simulink model "es1_catena_chiusa_2"  (R2014a)
settings: Solver=ode45  StartTime=0.0  StopTime=20.0  RelTol=1e-3
values from neighbouring files (symbols this model uses):
  Kc = 5    [es1.m]
libraries: cstblocks x2
settings Model: Creator=HP  LastModifiedBy=HP

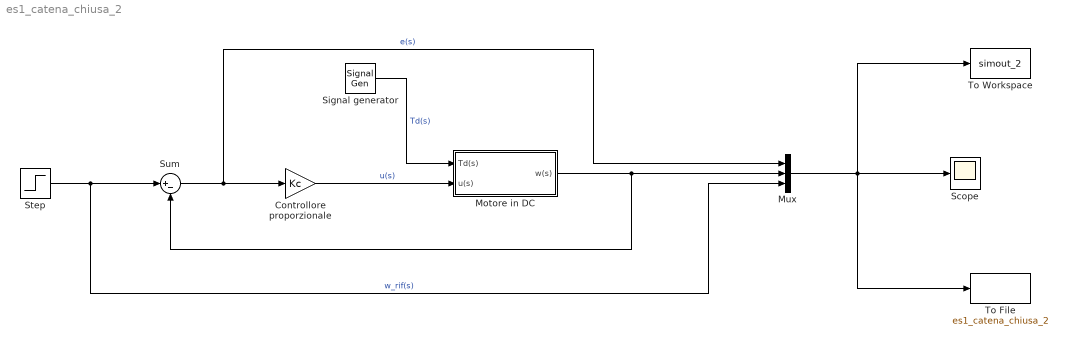
== system es1_catena_chiusa_2 ==
  Controllore proporzionale : Gain  Gain=Kc
  Motore in DC : Subsystem  TreatAsAtomicUnit=on
  Mux : Mux  Inputs=3
  Scope : Scope
      settings: MaxDataPoints=10000
  Signal generator : SignalGenerator  WaveForm=square  Amplitude=0.05  Frequency=0.1
  Step : Step  Time=0  SampleTime=0
  Sum : Sum  Inputs=|+-
  To File : ToFile  Filename=es1_catena_chiusa_2  MatrixName=output_2  SaveFormat=Timeseries
  To Workspace : ToWorkspace  VariableName=simout_2  SaveFormat=Timeseries  SampleTime=-1
  wires:
  Controllore proporzionale/1 -> Motore in DC/2(u(s))  "u(s)"
  Signal generator/1 -> Motore in DC/1(Td(s))  "Td(s)"
  Motore in DC/1(w(s)) -> Mux/2, Sum/2
  Step/1 -> Mux/3, Sum/1  "w_rif(s)"
  Sum/1 -> Mux/1, Controllore proporzionale/1  "e(s)"
  Mux/1 -> To File/1, Scope/1, To Workspace/1

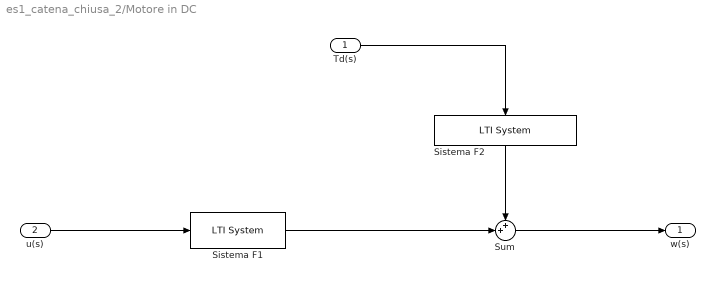
== system es1_catena_chiusa_2/Motore in DC ==
  Td(s) : Inport
  u(s) : Inport  Port=2
  Sistema F1 : cstblocks/LTI System  sys=F1  IC=[]
  Sistema F2 : cstblocks/LTI System  sys=F2  IC=[]
  Sum : Sum  Inputs=++|
  w(s) : Outport
  wires:
  u(s)/1 -> Sistema F1/1
  Sistema F2/1 -> Sum/1
  Sistema F1/1 -> Sum/2
  Sum/1 -> w(s)/1
  Td(s)/1 -> Sistema F2/1
